simulink model "E1a"  (R2017a)
settings: Solver=ode3  StartTime=0.0  StopTime=100.0  FixedStep=0.01  RelTol=1e-3
settings Model: Creator=Soutrik  LastModifiedBy=Soutrik

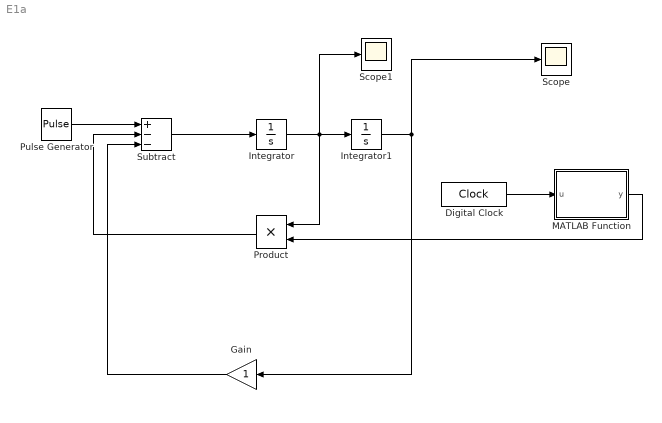
== system E1a ==
  Digital Clock : DigitalClock
  Gain : Gain
  Integrator : Integrator
  Integrator1 : Integrator
  MATLAB Function : MATLAB Function  TreatAsAtomicUnit=on
  Product : Product
  Pulse Generator : DiscretePulseGenerator  PulseType=Time based  Period=10  PulseWidth=50
  Scope : Scope
  Scope1 : Scope
  Subtract : Sum  Inputs=+--
  wires:
  Subtract/1 -> Integrator/1
  Pulse Generator/1 -> Subtract/1
  Gain/1 -> Subtract/3
  Product/1 -> Subtract/2
  Integrator/1 -> Scope1/1, Product/1, Integrator1/1
  Integrator1/1 -> Scope/1, Gain/1
  Digital Clock/1 -> MATLAB Function/1(u)
  MATLAB Function/1(y) -> Product/2

== matlab function E1a/MATLAB Function ==
  data: u input; y output
function y = fcn(u)
if u<24
    y=0.8;
else
    if u<55
        y=0.6;
    else
        if u<76
            y=0.4;
        else 
   
                y=0.2;
            
        end
    end
end

end
